simulink model "project_model"  (R2022b)
settings: Solver=VariableStepAuto  StartTime=0.0  StopTime=10.0  RelTol=1e-3
settings Model: Creator=yunuo  LastModifiedBy=yunuo

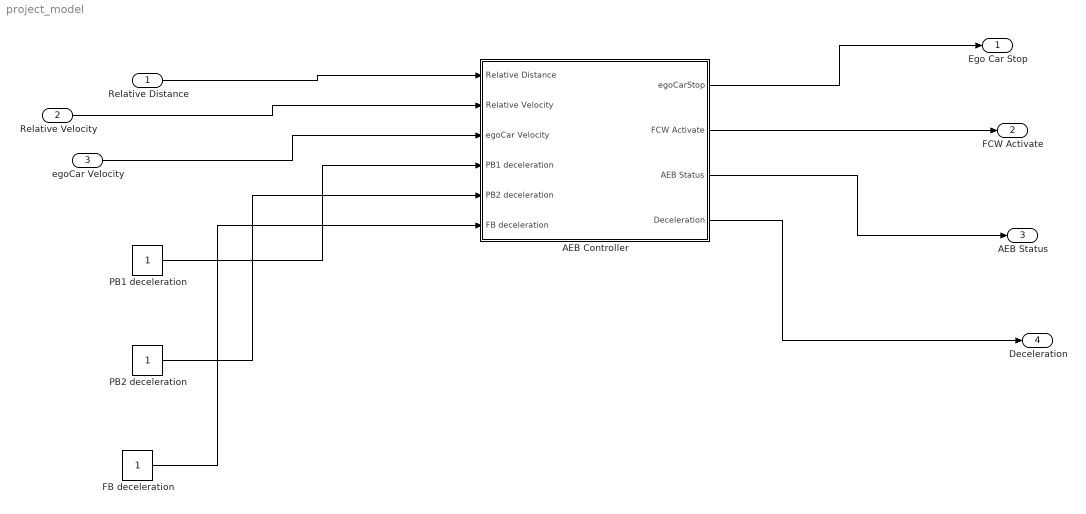
== system project_model ==
  Relative Distance : Inport
  Relative Velocity : Inport  Port=2
  egoCar Velocity : Inport  Port=3
  AEB Controller : Subsystem
  FB deceleration : Constant
  PB1 deceleration : Constant
  PB2 deceleration : Constant
  Ego Car Stop : Outport  PortDimensions=1  VectorParamsAs1DForOutWhenUnconnected=off
  FCW Activate : Outport  Port=2  OutDataTypeStr=uint8  PortDimensions=1  VectorParamsAs1DForOutWhenUnconnected=off
  AEB Status : Outport  Port=3  OutDataTypeStr=uint8  PortDimensions=1  VectorParamsAs1DForOutWhenUnconnected=off
  Deceleration : Outport  Port=4  OutDataTypeStr=uint8  PortDimensions=1  VectorParamsAs1DForOutWhenUnconnected=off
  wires:
  Relative Distance/1 -> AEB Controller/1(Relative Distance)
  Relative Velocity/1 -> AEB Controller/2(Relative Velocity)
  PB1 deceleration/1 -> AEB Controller/4(PB1 deceleration)
  PB2 deceleration/1 -> AEB Controller/5(PB2 deceleration)
  FB deceleration/1 -> AEB Controller/6(FB deceleration)
  egoCar Velocity/1 -> AEB Controller/3(egoCar Velocity)
  AEB Controller/1(egoCarStop) -> Ego Car Stop/1
  AEB Controller/2(FCW Activate) -> FCW Activate/1
  AEB Controller/3(AEB Status) -> AEB Status/1
  AEB Controller/4(Deceleration) -> Deceleration/1

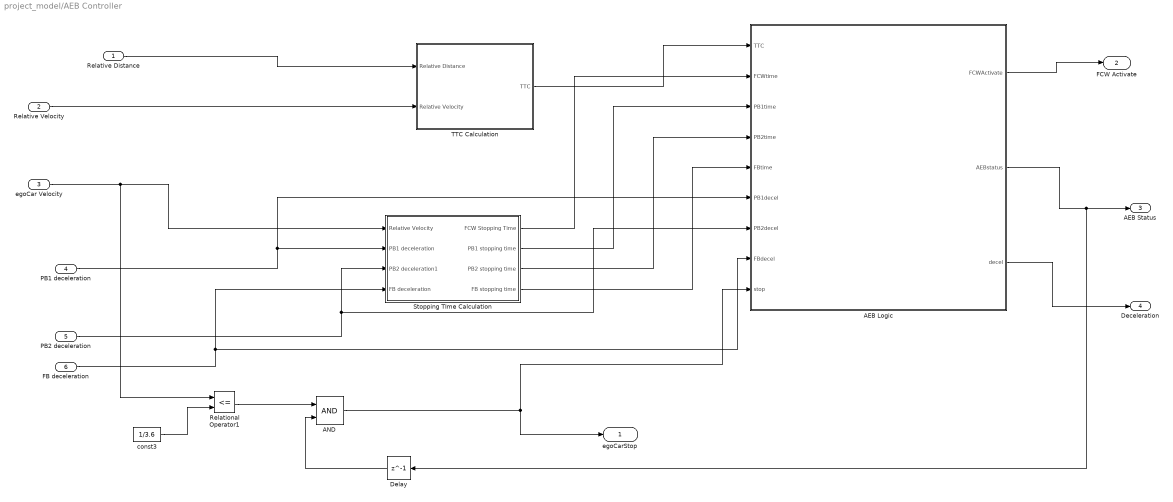
== system project_model/AEB Controller ==
  Relative Distance : Inport
  Relative Velocity : Inport  Port=2
  egoCar Velocity : Inport  Port=3
  PB1 deceleration : Inport  Port=4
  PB2 deceleration : Inport  Port=5
  FB deceleration : Inport  Port=6
  AEB Logic : Stateflow chart  TreatAsAtomicUnit=on
      settings: PortSchema="{\"entries\":[{\"content\":{\"sides\":[{\"content\":{\"connectorIds\":[\"In1\",\"In2\",\"In3\",\"In4\",\"In5\",\"In7\",\"In6\",\"In8\",\"In9\"]},\"type\":\"ConnectorPlacement.EquallySpacedRectSide\",\"uuid\":\"9d1a3049-a237-4f2f-9949-90932e1c60cf\"},{\"content\":{\"connectorIds\":[\"Out1\",\"Out2\",\"Out3\"],\"side\":\"RIGHT\"},\"type\":\"ConnectorPlacement.EquallySpacedRectSide\",\"uuid\":\"cbd9d543-c0a7-4fd7-9ff9-23f2589f349f\"},{\"content\":{\"connectorIds\":[],\"side\":\"TOP\"},\"type\":\"ConnectorPlacement.EquallySpacedRectSide\",\"uuid\":\"e3d4d77f-c8bb-4ad5-a2ee-6e300ca59f69\"}]},\"type\":\"ConnectorPlacement.EquallySpacedConnector\",\"uuid\":\"64ee3bf6-4fd0-4aa2-b421-1dac464e21b4\"}],\"packageUris\":[\"http://schema.mathworks.com/mf0/Connector/R2020b\"],\"version\":\"1.0\"}"
  AND : Logic  IconShape=distinctive  AllPortsSameDT=off  OutDataTypeStr=boolean
  Delay : Delay  DelayLength=1
  Relational Operator1 : RelationalOperator  Operator=<=  OutDataTypeStr=boolean  RndMeth=Simplest  InputSameDT=off
  Stopping TIme Calculation : Subsystem
  TTC Calculation : Subsystem
  const3 : Constant  Value=1/3.6  SampleTime=-1
  egoCarStop : Outport  VectorParamsAs1DForOutWhenUnconnected=off
  FCW Activate : Outport  Port=2  VectorParamsAs1DForOutWhenUnconnected=off
  AEB Status : Outport  Port=3  VectorParamsAs1DForOutWhenUnconnected=off
  Deceleration : Outport  Port=4  OutDataTypeStr=double  VectorParamsAs1DForOutWhenUnconnected=off
  wires:
  Relative Distance/1 -> TTC Calculation/1(Relative Distance)
  Relative Velocity/1 -> TTC Calculation/2(Relative Velocity)
  PB1 deceleration/1 -> AEB Logic/7(PB1decel), Stopping TIme Calculation/2(PB1 deceleration)
  PB2 deceleration/1 -> AEB Logic/6(PB2decel), Stopping TIme Calculation/3(PB2 deceleration1)
  FB deceleration/1 -> AEB Logic/8(FBdecel), Stopping TIme Calculation/4(FB deceleration)
  TTC Calculation/1(TTC) -> AEB Logic/1(TTC)
  Stopping TIme Calculation/1(FCW Stopping Time) -> AEB Logic/2(FCWtime)
  Stopping TIme Calculation/2(PB1 stopping time) -> AEB Logic/3(PB1time)
  Stopping TIme Calculation/3(PB2 stopping time) -> AEB Logic/4(PB2time)
  Stopping TIme Calculation/4(FB stopping time) -> AEB Logic/5(FBtime)
  const3/1 -> Relational Operator1/2
  egoCar Velocity/1 -> Relational Operator1/1, Stopping TIme Calculation/1(Relative Velocity)
  Relational Operator1/1 -> AND/1
  AND/1 -> egoCarStop/1, AEB Logic/9(stop)
  Delay/1 -> AND/2
  AEB Logic/1(FCWActivate) -> FCW Activate/1
  AEB Logic/2(AEBstatus) -> Delay/1, AEB Status/1
  AEB Logic/3(decel) -> Deceleration/1

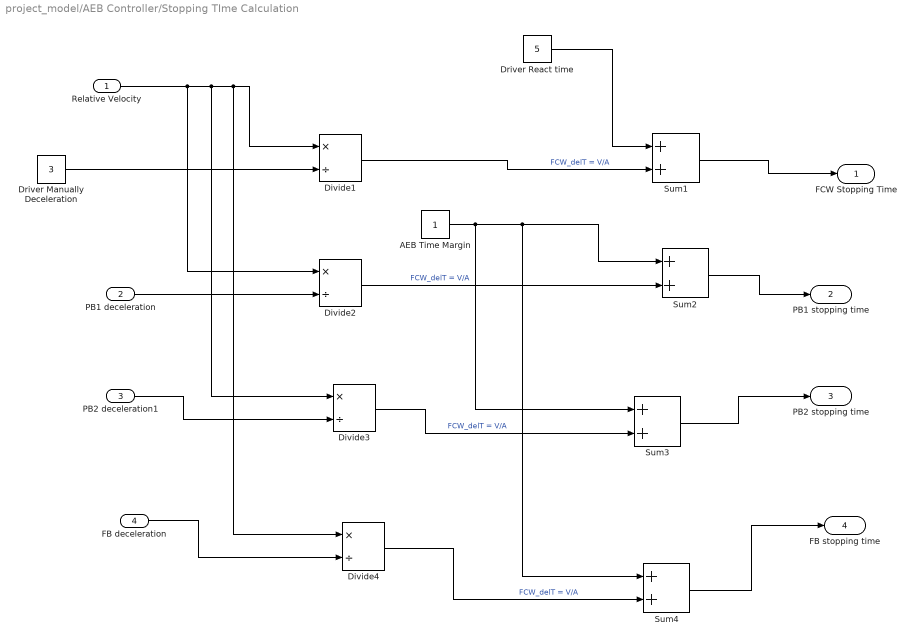
== system project_model/AEB Controller/Stopping TIme Calculation ==
  Relative Velocity : Inport
  PB1 deceleration : Inport  Port=2
  PB2 deceleration1 : Inport  Port=3
  FB deceleration : Inport  Port=4
  AEB Time Margin : Constant
  Divide{1..4} (4 alike) : Product  Inputs=*/
  Driver Manually Deceleration : Constant  Value=3
  Driver React time : Constant  Value=5
  Sum{1..4} (4 alike) : Sum
  FCW Stopping Time : Outport
  PB1 stopping time : Outport  Port=2
  PB2 stopping time : Outport  Port=3
  FB stopping time : Outport  Port=4
  wires:
  Relative Velocity/1 -> Divide4/1, Divide1/1, Divide3/1, Divide2/1
  Driver Manually Deceleration/1 -> Divide1/2
  Divide1/1 -> Sum1/2  "FCW_delT = V/A"
  Driver React time/1 -> Sum1/1
  Sum1/1 -> FCW Stopping Time/1
  PB1 deceleration/1 -> Divide2/2
  PB2 deceleration1/1 -> Divide3/2
  FB deceleration/1 -> Divide4/2
  Divide2/1 -> Sum2/2  "FCW_delT = V/A"
  AEB Time Margin/1 -> Sum3/1, Sum4/1, Sum2/1
  Divide3/1 -> Sum3/2  "FCW_delT = V/A"
  Divide4/1 -> Sum4/2  "FCW_delT = V/A"
  Sum2/1 -> PB1 stopping time/1
  Sum3/1 -> PB2 stopping time/1
  Sum4/1 -> FB stopping time/1

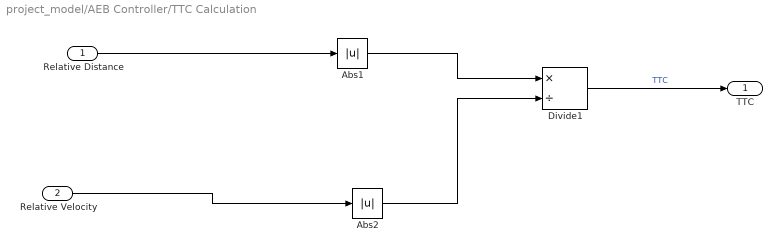
== system project_model/AEB Controller/TTC Calculation ==
  Relative Distance : Inport
  Relative Velocity : Inport  Port=2
  Abs1 : Abs  SaturateOnIntegerOverflow=off
  Abs2 : Abs  SaturateOnIntegerOverflow=off
  Divide1 : Product  Inputs=*/
  TTC : Outport
  wires:
  Divide1/1 -> TTC/1  "TTC"
  Abs1/1 -> Divide1/1
  Abs2/1 -> Divide1/2
  Relative Distance/1 -> Abs1/1
  Relative Velocity/1 -> Abs2/1

== stateflow chart project_model/AEB Controller/AEB Logic ==
  state Default
    entry: AEBstatus = 0;
    FCWactivate = 0;
    decel = 0;
  state FCW
    entry: AEBstatus = 0;
    FCWactivate = 1;
    decel = 0;
  state Partial_Braking1
    entry: AEBstatus = 1;
    FCWactivate = 1;
    decel = PB1decel;
  state Full_Braking
    entry: AEBstatus = 3;
    FCWactivate = 1;
    decel = FBdecel;
  state Partial_Braking2
    entry: AEBstatus = 2;
    FCWactivate = 1;
    decel = PB2decel;
  (default) -> Default
  Full_Braking -> Default : [stop==1]
  Partial_Braking2 -> Default [order 2] : [stop==1]
  Partial_Braking1 -> Default [order 2] : [stop==1]
  Default -> FCW : [(abs(TTC)<FCWtime) && TTC<0]
  FCW -> Default [order 2] : [abs(TTC)>=1.2*FCWtime]
  FCW -> Partial_Braking1 [order 1] : [(abs(TTC) < PB1time) && TTC<0]
  Partial_Braking1 -> Partial_Braking2 [order 1] : [(abs(TTC) < PB2time) && TTC<0]
  Partial_Braking2 -> Full_Braking [order 1] : [(abs(TTC) < FBtime) && TTC<0]
  data: TTC input; FCWtime input; PB1time input; PB2time input; FBtime input; PB2decel input; PB1decel input; FBdecel input; stop input; FCWActivate output; AEBstatus output; decel output
